simulink model "lab3kalman"  (R2018a)
settings: Solver=VariableStepAuto  StartTime=0.0  StopTime=5  RelTol=1e-3
values from neighbouring files (symbols this model uses):
  hf = tf(0.2, [150, 53, 1], 'iodelay', 2)    [lab3ex2.m]
  hrz = tf((1-exp(-T/lambda))*[1, a1, a2, 0],     [(b1+b2), -(b1+b2)*exp(-T/lambda), 0, -b1*(1-exp(-T/lambda))-b2*(1-exp(-T/lambda))], T)    [lab3ex2.m]
  T = 1    [lab3ex2.m]
settings Model: Creator=User  LastModifiedBy=User

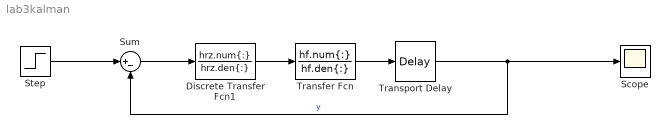
== system lab3kalman ==
  Discrete Transfer Fcn1 : DiscreteTransferFcn  Numerator=hrz.num{:}  Denominator=hrz.den{:}  SampleTime=T
  Scope : Scope
  Step : Step  Time=0  SampleTime=0
  Sum : Sum  Inputs=|+-
  Transfer Fcn : TransferFcn  Numerator=hf.num{:}  Denominator=hf.den{:}
  Transport Delay : TransportDelay  DelayTime=1.86
  wires:
  Sum/1 -> Discrete Transfer Fcn1/1
  Transport Delay/1 -> Sum/2, Scope/1  "y"
  Step/1 -> Sum/1
  Discrete Transfer Fcn1/1 -> Transfer Fcn/1
  Transfer Fcn/1 -> Transport Delay/1
